simulink model "mseExampleDelayWithCase"  (R2023b)
settings: Solver=VariableStepAuto  StartTime=0.0  StopTime=20  FixedStep=1  MaxStep=.1  RelTol=1e-3
libraries: simulink x1
settings Model: PacingRate=0.110000  Creator=DarianMuresan  LastModifiedBy=DarianMuresan

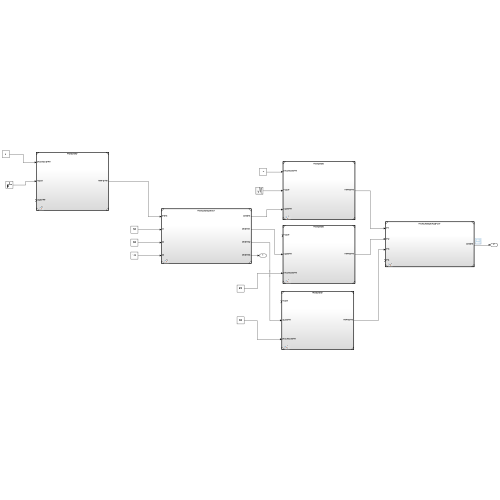
[thumbnail: Simulink's stored preview of the top-level diagram]
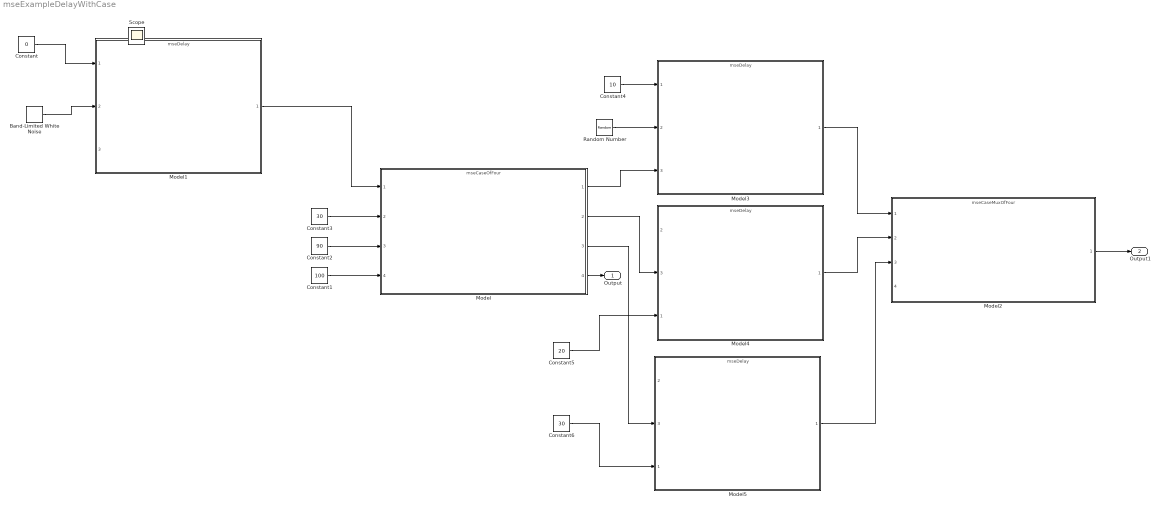
== system mseExampleDelayWithCase ==
  Band-Limited White Noise : simulink/Sources/Band-Limited White Noise  Cov=0.01  Ts=0.1  seed=[23341]
  Constant : Constant  Value=0
  Constant1 : Constant  Value=100
  Constant2 : Constant  Value=90
  Constant3 : Constant  Value=30
  Constant4 : Constant  Value=10
  Constant5 : Constant  Value=20
  Constant6 : Constant  Value=30
  Model : ModelReference  ModelNameDialog=mseCaseOfFour.slx  SimulationMode=Normal  ModelReferenceVersion=1.14
  Model{1,3..5} (4 alike) : ModelReference  ModelNameDialog=mseDelay.slx  SimulationMode=Normal  ModelReferenceVersion=1.7
      Model4 settings: PortSchema="{\"entries\":[{\"content\":{\"sides\":[{\"content\":{\"connectorIds\":[\"In2\",\"In3\",\"In1\"]},\"type\":\"ConnectorPlacement.EquallySpacedRectSide\",\"uuid\":\"49f3e86f-0adf-41fc-85ec-5be0cbef3cd0\"},{\"content\":{\"connectorIds\":[\"Out1\"],\"side\":\"RIGHT\"},\"type\":\"ConnectorPlacement.EquallySpacedRectSide\",\"uuid\":\"012fc00d-9423-4eca-973e-f184ade09ed6\"},{\"content\":{\"side\":\"TOP\"},\"type\":\"ConnectorPlacement.EquallySpacedRectSide\",\"uuid\":\"5f09439f-c95e-472b-a3b3-847b37323f3c\"}]},\"type\":\"ConnectorPlacement.EquallySpacedConnector\",\"uuid\":\"443a1937-b1b0-43b8-bfc0-210971d96f52\"}],\"packageUris\":[\"http://schema.mathworks.com/mf0/Connector/R2020b\"],\"version\":\"1.0\"}"
      Model5 settings: PortSchema="{\"entries\":[{\"content\":{\"sides\":[{\"content\":{\"connectorIds\":[\"In2\",\"In3\",\"In1\"]},\"type\":\"ConnectorPlacement.EquallySpacedRectSide\",\"uuid\":\"49f3e86f-0adf-41fc-85ec-5be0cbef3cd0\"},{\"content\":{\"connectorIds\":[\"Out1\"],\"side\":\"RIGHT\"},\"type\":\"ConnectorPlacement.EquallySpacedRectSide\",\"uuid\":\"012fc00d-9423-4eca-973e-f184ade09ed6\"},{\"content\":{\"side\":\"TOP\"},\"type\":\"ConnectorPlacement.EquallySpacedRectSide\",\"uuid\":\"5f09439f-c95e-472b-a3b3-847b37323f3c\"}]},\"type\":\"ConnectorPlacement.EquallySpacedConnector\",\"uuid\":\"443a1937-b1b0-43b8-bfc0-210971d96f52\"}],\"packageUris\":[\"http://schema.mathworks.com/mf0/Connector/R2020b\"],\"version\":\"1.0\"}"
  Model2 : ModelReference  ModelNameDialog=mseCaseMuxOfFour.slx  SimulationMode=Normal  ModelReferenceVersion=1.5
  Random Number : RandomNumber  Variance=0.2  SampleTime=0.1
  Output : Outport
  Output1 : Outport  Port=2
  Scope : Scope
  wires:
  Constant/1 -> Model1/1
  Constant1/1 -> Model/4
  Constant2/1 -> Model/3
  Constant3/1 -> Model/2
  Model1/1 -> Model/1
  Model/1 -> Model3/3
  Model/4 -> Output/1
  Constant4/1 -> Model3/1
  Model/2 -> Model4/3
  Model/3 -> Model5/3
  Constant5/1 -> Model4/1
  Constant6/1 -> Model5/1
  Model3/1 -> Model2/1
  Model4/1 -> Model2/2
  Model5/1 -> Model2/3
  Model2/1 -> Output1/1
  Band-Limited White Noise/1 -> Model1/2
  Random Number/1 -> Model3/2
